simulink model "stateflow_0"  (R2021b)
settings: Solver=VariableStepAuto  StartTime=0.0  StopTime=10.0  RelTol=1e-3
settings Model: Creator=fredric  LastModifiedBy=fredric

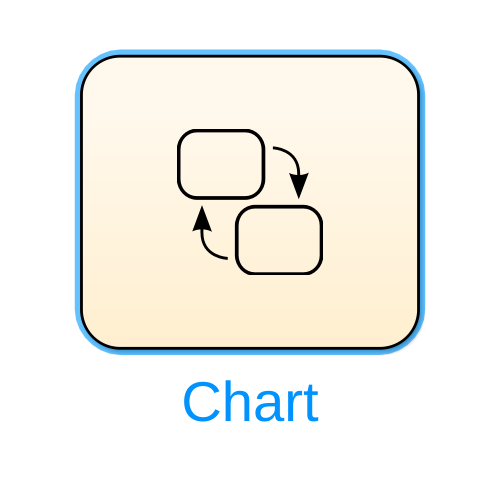
[thumbnail: Simulink's stored preview of the top-level diagram]
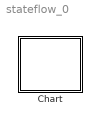
== system stateflow_0 ==
  Chart : Stateflow chart  TreatAsAtomicUnit=on

== stateflow chart stateflow_0/Chart ==
  (default) -> (junction 1)
  (junction 1) -> (junction 3) [order 1] : [ input == 1 ]
  (junction 1) -> (junction 9) [order 2] : {
      |    output =  0;
      | }
  (junction 3) -> (junction 7) : {
      |     output = 2;
      | }
  (junction 7) -> (junction 9)
  (junction 9) -> (junction 11)
